simulink model "Perfect_Lineaer"  (R2017a)
settings: Solver=VariableStepAuto  StartTime=0.0  StopTime=17  FixedStep=0.01  RelTol=1e-3
values from neighbouring files (symbols this model uses):
  A = [-4.65E-06	0.0001701	-0.0002836	0	0	0	-2.56E-06	-7.97E-06	3.61E-06 ... (first row only)    [surfaces_setup_test.m]
  A0 = [-4.65E-06	0.0001701	-0.0002836	0	0	0	0	-1.43	0 ... (first row only)    [surfaces_setup_test.m]
  a0_s2345 = [0;0;0.05;0.05]    [HW5_4_surfaces.m]    (also in TEST_aerosetup.m; surfaces_setup_test.m)
  A_2345 = c_2345.*b_2345    [HW5_4_surfaces.m]    (also in TEST_aerosetup.m; surfaces_setup_test.m)
  Aileron_left = 0    [HW5_4_surfaces.m]    (also in TEST_aerosetup.m; surfaces_setup_test.m)
  Aileron_right = 0    [HW5_4_surfaces.m]    (also in TEST_aerosetup.m; surfaces_setup_test.m)
  B = [-7.98E-09	7.83E-09	1.68E-09	2.75E-10 ... (first row only)    [surfaces_setup_test.m]
  B0 = [-6.2	6.2	0	0.45 ... (first row only)    [surfaces_setup_test.m]
  c_2345 = [0.075;0.08;0.1;0.1]    [HW5_4_surfaces.m]    (also in TEST_aerosetup.m; surfaces_setup_test.m)
  CD0_s2345 = [0.01;0.01;0.01;0.01]    [HW5_4_surfaces.m]    (also in TEST_aerosetup.m; surfaces_setup_test.m)
  CDa_s2345 = [1;1;1;1]    [HW5_4_surfaces.m]    (also in TEST_aerosetup.m; surfaces_setup_test.m)
  CL0_2345 = [0;0; 0.05; 0.05]    [HW5_4_surfaces.m]    (also in TEST_aerosetup.m; surfaces_setup_test.m)
  CLa = 2*pi*(r./(2+r))    [HW5_4_surfaces.m]    (also in TEST_aerosetup.m; surfaces_setup_test.m)
  CM0_s2345 = [0;0;-0.05;-0.05]    [HW5_4_surfaces.m]    (also in TEST_aerosetup.m; surfaces_setup_test.m)
  CMa_s2345 = [0; 0; 0; 0]    [HW5_4_surfaces.m]    (also in TEST_aerosetup.m; surfaces_setup_test.m)
  e_s2345 = [0.8;0.8;0.9;0.9]    [HW5_4_surfaces.m]    (also in TEST_aerosetup.m; surfaces_setup_test.m)
  elevator = 0    [HW5_4_surfaces.m]    (also in TEST_aerosetup.m; surfaces_setup_test.m)
  Fext_N = -g_EN * m    [HW5_4_surfaces.m]    (also in TEST_aerosetup.m = [10 10 10]; surfaces_setup_test.m)
  g_EN = [0; 0; 9.81]    [HW5_4_surfaces.m]    (also in TEST_aerosetup.m = [0; 0; 9.8]; surfaces_setup_test.m)
  i_s2345 = [0; 0; 0.05; 0.05;]    [HW5_4_surfaces.m]    (also in TEST_aerosetup.m; surfaces_setup_test.m)
  J_cgp = ones(3)    [surfaces_setup_test.m]
  M_total = sum(MnG(:,1))/1000    [HW5_4_surfaces.m]    (also in TEST_aerosetup.m; surfaces_setup_test.m = sum(MnG1(:,1))/1000)
  Mext_B = [0; 0; 0]    [HW5_4_surfaces.m]    (also in TEST_aerosetup.m = [1; 1; 1]; surfaces_setup_test.m)
  p_E_BE_ini = p_E_BE_ini_deg .* [deg2rad; deg2rad; 1]    [HW5_4_surfaces.m]    (also in TEST_aerosetup.m; surfaces_setup_test.m)
  r = b_2345./c_2345    [HW5_4_surfaces.m]    (also in TEST_aerosetup.m; surfaces_setup_test.m)
  Rearth = 6371000    [HW5_4_surfaces.m]    (also in TEST_aerosetup.m; surfaces_setup_test.m)
  rudder = 0    [HW5_4_surfaces.m]    (also in TEST_aerosetup.m; surfaces_setup_test.m)
  Theta_ini = Theta_ini_deg * deg2rad    [HW5_4_surfaces.m]    (also in TEST_aerosetup.m; surfaces_setup_test.m)
  U0 = [Aileron_right;Aileron_left;elevator;rudder]    [surfaces_setup_test.m]
  v_N_AE = [0;0;0]    [HW5_4_surfaces.m]    (also in TEST_aerosetup.m; surfaces_setup_test.m)
  Vbbe_int = [10; 0; 0]    [HW5_4_surfaces.m]    (also in TEST_aerosetup.m; surfaces_setup_test.m = [5; 0; 0])
  w_B_BE_ini = [1e0; 1e-2; 1e-2]    [HW5_4_surfaces.m]    (also in TEST_aerosetup.m; surfaces_setup_test.m)
  X0 = [w_B_BE_ini;Theta_ini;Vbbe_int]    [surfaces_setup_test.m]
  xyz_s = [[-0.76 0 0.16];[-0.76 0 -0.09];[-0.23 0.44 0];[-0.23 -0.44 0];]    [HW5_4_surfaces.m]    (also in TEST_aerosetup.m; surfaces_setup_test.m)
undefined symbols (not defined in the file or in its folder): Discrete, Earth, K, Time, WGS84
libraries: simulink x83, aerolibfltsims x5, dspsrcs4 x4, simulink_extras x4, dspinverses x3, vrlib x2, sharedtransform x1, aerolibtransform2 x1, aerolibutil x1, sharedutil x1, ctrlSharedLib x1
(part 2 of 8)

== system Perfect_Lineaer/My State Equa_with surf ==
  Band-Limited White Noise : simulink/Sources/Band-Limited White Noise  Cov=[0.1]  Ts=0.1  seed=[23341]
  Colored Noise : dspsrcs4/Colored Noise  Color=white  InverseFrequencyPower=1  NumChannels=1  OutputDataType=double  SamplesPerFrame=1  SampleTime=0.001  RandomStream=mt19937ar with seed  Seed=67  SimulateUsing=Interpreted execution
      settings: SourceProductName=DSP System Toolbox  SourceProductBaseCode=DS
  Demux : Demux  Outputs=3  BusSelectionMode=on
  Demux1 : Demux  Outputs=3
  Demux2 : Demux  Outputs=3
  Gain : Gain
  Gain1 : Gain  Gain=0.05
  Gain2 : Gain  Gain=0.01
  Mux1 : Mux  Inputs=2
  Mux2 : Mux  Inputs=2
  Mux3 : Mux  Inputs=2
  PID Controller : simulink/Continuous/PID Controller  Controller=PID  TimeDomain=Continuous-time  SampleTime=-1  IntegratorMethod=Forward Euler  FilterMethod=Forward Euler  Form=Parallel  UseFilter=on  ControllerParametersSource=internal  P=-1.24371882307401e-06  I=-2.52279405780551e-11  D=-0.0136233397121708  N=0.397355587236386  InitialConditionSource=internal  InitialConditionForIntegrator=0  InitialConditionForFilter=0  ExternalReset=none  LimitOutput=off  UpperSaturationLimit=inf  LowerSaturationLimit=-inf  LinearizeAsGain=on  AntiWindupMode=none  Kb=1  TrackingMode=off  Kt=1  PParamMin=[]  PParamMax=[]  IParamMin=[]  IParamMax=[]  DParamMin=[]  DParamMax=[]  NParamMin=[]  NParamMax=[]  KbParamMin=[]  KbParamMax=[]  KtParamMin=[]  KtParamMax=[]  POutMin=[]  POutMax=[]  IOutMin=[]  IOutMax=[]  DOutMin=[]  DOutMax=[]  NOutMin=[]  NOutMax=[]  KbOutMin=[]  KbOutMax=[]  KtOutMin=[]  KtOutMax=[]  IntegratorOutMin=[]  IntegratorOutMax=[]  FilterOutMin=[]  FilterOutMax=[]  SumOutMin=[]  SumOutMax=[]  SumI1OutMin=[]  SumI1OutMax=[]  SumI2OutMin=[]  SumI2OutMax=[]  SumI3OutMin=[]  SumI3OutMax=[]  SumDOutMin=[]  SumDOutMax=[]  SaturationOutMin=[]  SaturationOutMax=[]  IntegratorContinuousStateAttributes=''  IntegratorStateMustResolveToSignalObject=off  IntegratorRTWStateStorageClass=Auto  FilterContinuousStateAttributes=''  FilterStateMustResolveToSignalObject=off  FilterRTWStateStorageClass=Auto  DifferentiatorICPrevScaledInput=0  DifferentiatorOutMin=[]  DifferentiatorOutMax=[]  InitialConditionSetting=State (most efficient)
  PID Controller1 : simulink/Continuous/PID Controller  Controller=PID  TimeDomain=Continuous-time  SampleTime=-1  IntegratorMethod=Forward Euler  FilterMethod=Forward Euler  Form=Parallel  UseFilter=on  ControllerParametersSource=internal  P=0.206020341004349  I=0.0106225881647426  D=0.887791188699333  N=1010.04325893263  InitialConditionSource=internal  InitialConditionForIntegrator=0  InitialConditionForFilter=0  ExternalReset=none  LimitOutput=off  UpperSaturationLimit=inf  LowerSaturationLimit=-inf  LinearizeAsGain=on  AntiWindupMode=none  Kb=1  TrackingMode=off  Kt=1  PParamMin=[]  PParamMax=[]  IParamMin=[]  IParamMax=[]  DParamMin=[]  DParamMax=[]  NParamMin=[]  NParamMax=[]  KbParamMin=[]  KbParamMax=[]  KtParamMin=[]  KtParamMax=[]  POutMin=[]  POutMax=[]  IOutMin=[]  IOutMax=[]  DOutMin=[]  DOutMax=[]  NOutMin=[]  NOutMax=[]  KbOutMin=[]  KbOutMax=[]  KtOutMin=[]  KtOutMax=[]  IntegratorOutMin=[]  IntegratorOutMax=[]  FilterOutMin=[]  FilterOutMax=[]  SumOutMin=[]  SumOutMax=[]  SumI1OutMin=[]  SumI1OutMax=[]  SumI2OutMin=[]  SumI2OutMax=[]  SumI3OutMin=[]  SumI3OutMax=[]  SumDOutMin=[]  SumDOutMax=[]  SaturationOutMin=[]  SaturationOutMax=[]  IntegratorContinuousStateAttributes=''  IntegratorStateMustResolveToSignalObject=off  IntegratorRTWStateStorageClass=Auto  FilterContinuousStateAttributes=''  FilterStateMustResolveToSignalObject=off  FilterRTWStateStorageClass=Auto  DifferentiatorICPrevScaledInput=0  DifferentiatorOutMin=[]  DifferentiatorOutMax=[]  InitialConditionSetting=State (most efficient)
  PID Controller2 : simulink/Continuous/PID Controller  Controller=PID  TimeDomain=Continuous-time  SampleTime=-1  IntegratorMethod=Forward Euler  FilterMethod=Forward Euler  Form=Parallel  UseFilter=on  ControllerParametersSource=internal  P=0.206020341004349  I=0.0106225881647426  D=0.887791188699333  N=1010.04325893263  InitialConditionSource=internal  InitialConditionForIntegrator=0  InitialConditionForFilter=0  ExternalReset=none  LimitOutput=off  UpperSaturationLimit=inf  LowerSaturationLimit=-inf  LinearizeAsGain=on  AntiWindupMode=none  Kb=1  TrackingMode=off  Kt=1  PParamMin=[]  PParamMax=[]  IParamMin=[]  IParamMax=[]  DParamMin=[]  DParamMax=[]  NParamMin=[]  NParamMax=[]  KbParamMin=[]  KbParamMax=[]  KtParamMin=[]  KtParamMax=[]  POutMin=[]  POutMax=[]  IOutMin=[]  IOutMax=[]  DOutMin=[]  DOutMax=[]  NOutMin=[]  NOutMax=[]  KbOutMin=[]  KbOutMax=[]  KtOutMin=[]  KtOutMax=[]  IntegratorOutMin=[]  IntegratorOutMax=[]  FilterOutMin=[]  FilterOutMax=[]  SumOutMin=[]  SumOutMax=[]  SumI1OutMin=[]  SumI1OutMax=[]  SumI2OutMin=[]  SumI2OutMax=[]  SumI3OutMin=[]  SumI3OutMax=[]  SumDOutMin=[]  SumDOutMax=[]  SaturationOutMin=[]  SaturationOutMax=[]  IntegratorContinuousStateAttributes=''  IntegratorStateMustResolveToSignalObject=off  IntegratorRTWStateStorageClass=Auto  FilterContinuousStateAttributes=''  FilterStateMustResolveToSignalObject=off  FilterRTWStateStorageClass=Auto  DifferentiatorICPrevScaledInput=0  DifferentiatorOutMin=[]  DifferentiatorOutMax=[]  InitialConditionSetting=State (most efficient)
  Scope{,1..4} (5 alike) : Scope
  State-Space (with initial outputs) : simulink_extras/Additional Linear/State-Space (with initial outputs)  A=|  B=[1;1;1;1;1;1;1;1;1]  C=eye(9)  D=[0;0;0;0;0;0;0;0;0]  U0=1  Y0=.5
      | [4.65E-06	0.0003206	-0.0002836	0	0	0	-3.61E-06	-1.11E-05	5.08E-06;
      | -0.0004817	0	0.004483	0	0	0	-0.0009403	0.0007193	-0.001111;
      | 0.0001102	0.001788	-4.65E-06	0	0	0	-4.49E-05	-0.000135	6.27E-05;
      | 1	0.3858	-0.8841	-0.0001586	0.0006637	0	0	0	0;
      | 0	-0.9165	-0.3999	-0.0003438	0	0	0	0	0;
      | 0	0.5557	-1.273	-0.0002285	0.0004608	0	0	0	0;
      | 0	-0.003349	0.002001	-3.476	-2.786	3.102	0.0001527	-0.0002979	-0.0001301;
      | 0.003349	0	0.002582	-30.67	-2.13	30.73	0.0002746	7.64E-05	0.00463;
      | -0.002001	-0.002582	0	-1.42E-10	-22.26	-3.329	0.0001314	-0.004547	-0.0001848
      | ]
      settings: SourceProductName=Simulink  SourceProductBaseCode=SL
  State-Space (with initial outputs)1 : simulink_extras/Additional Linear/State-Space (with initial outputs)  A=|  B=[1;1;1]  C=eye(3)  D=[0;0;0]  U0=1  Y0=.5
      | [0	0.01	0;
      | -0.01	0	0;
      | 0.01	0	0
      | ]
      settings: SourceProductName=Simulink  SourceProductBaseCode=SL
  State-Space (with initial outputs)2 : simulink_extras/Additional Linear/State-Space (with initial outputs)  A=|  B=[1;1;1;1]  C=eye(4)  D=[0;0;0;0]  U0=1  Y0=.5
      | [-0.0025	0.4999	0.004999	0.0025;
      | -0.2475	0	0.004999	0.2475;
      | -0.2524	-0.004999	0	0.2524;
      | -0.0025	0.004999	-0.4999	0.0025
      | ]
      settings: SourceProductName=Simulink  SourceProductBaseCode=SL
  Step1 : Step  Time=5  After=-50  SampleTime=0
  Step2 : Step  Time=5  After=-50  SampleTime=0
  Step3 : Step  Time=5  After=-50  SampleTime=0
  Sum : Sum  Inputs=|+-
  Sum1 : Sum  Inputs=|+++
  Sum2 : Sum  Inputs=|+-
  Sum3 : Sum  Inputs=|+-
  Terminator{,1..5} (6 alike) : Terminator
  wires:
  Step3/1 -> Mux1/2, Sum/1
  Mux1/1 -> Scope1/1
  Sum/1 -> PID Controller/1
  Demux/2 -> Terminator1/1
  Demux/1 -> Terminator/1
  Demux/3 -> Sum1/1, Mux1/1
  State-Space (with initial outputs)/1 -> Scope2/1, Demux/1
  Colored Noise/1 -> Sum1/2
  PID Controller/1 -> State-Space (with initial outputs)/1
  Sum1/1 -> Gain/1
  Gain/1 -> Sum/2, Scope/1
  Band-Limited White Noise/1 -> Sum1/3
  Demux2/1 -> Terminator4/1
  Mux3/1 -> Scope4/1
  Demux2/3 -> Mux3/1, Gain2/1
  State-Space (with initial outputs)1/1 -> Demux1/1
  Mux2/1 -> Scope3/1
  Step2/1 -> Mux2/2, Sum2/1
  Step1/1 -> Mux3/2, Sum3/1
  Sum3/1 -> PID Controller2/1
  Demux1/2 -> Terminator3/1
  Demux1/3 -> Mux2/1, Gain1/1
  Gain2/1 -> Sum3/2
  Demux2/2 -> Terminator5/1
  PID Controller2/1 -> State-Space (with initial outputs)2/1
  Gain1/1 -> Sum2/2
  PID Controller1/1 -> State-Space (with initial outputs)1/1
  Sum2/1 -> PID Controller1/1
  Demux1/1 -> Terminator2/1
  State-Space (with initial outputs)2/1 -> Demux2/1

== system Perfect_Lineaer/Perfect_State Equa ==
  note: Inner loop
  note: Outer loop
  note: State loop
  A0 : Gain  Gain=A0  Multiplication=Matrix(K*u)
  B0 : Gain  Gain=B0  Multiplication=Matrix(K*u)
  Band-Limited White Noise : simulink/Sources/Band-Limited White Noise  Commented=on  Cov=[0.1]  Ts=0.1  seed=[23341]
  Colored Noise : dspsrcs4/Colored Noise  Commented=on  Color=white  InverseFrequencyPower=1  NumChannels=1  OutputDataType=double  SamplesPerFrame=1  SampleTime=0.001  RandomStream=mt19937ar with seed  Seed=67  SimulateUsing=Interpreted execution
      settings: SourceProductName=DSP System Toolbox  SourceProductBaseCode=DS
  Constant : Constant  Value=U0
  Constant1 : Constant  Value=X0
  Integrator : Integrator  InitialConditionSource=external
  Kd Based on Rlocus : Gain  Multiplication=Matrix(K*u)
  Kp for speed control : Gain  Commented=on
  PID Controller : simulink/Continuous/PID Controller  Controller=PID  TimeDomain=Continuous-time  SampleTime=-1  IntegratorMethod=Forward Euler  FilterMethod=Forward Euler  Form=Parallel  UseFilter=on  ControllerParametersSource=internal  P=10  I=0  D=0  N=100  InitialConditionSource=internal  InitialConditionForIntegrator=0  InitialConditionForFilter=0  ExternalReset=none  LimitOutput=off  UpperSaturationLimit=inf  LowerSaturationLimit=-inf  LinearizeAsGain=on  AntiWindupMode=none  Kb=1  TrackingMode=off  Kt=1  PParamMin=[]  PParamMax=[]  IParamMin=[]  IParamMax=[]  DParamMin=[]  DParamMax=[]  NParamMin=[]  NParamMax=[]  KbParamMin=[]  KbParamMax=[]  KtParamMin=[]  KtParamMax=[]  POutMin=[]  POutMax=[]  IOutMin=[]  IOutMax=[]  DOutMin=[]  DOutMax=[]  NOutMin=[]  NOutMax=[]  KbOutMin=[]  KbOutMax=[]  KtOutMin=[]  KtOutMax=[]  IntegratorOutMin=[]  IntegratorOutMax=[]  FilterOutMin=[]  FilterOutMax=[]  SumOutMin=[]  SumOutMax=[]  SumI1OutMin=[]  SumI1OutMax=[]  SumI2OutMin=[]  SumI2OutMax=[]  SumI3OutMin=[]  SumI3OutMax=[]  SumDOutMin=[]  SumDOutMax=[]  SaturationOutMin=[]  SaturationOutMax=[]  IntegratorContinuousStateAttributes=''  IntegratorStateMustResolveToSignalObject=off  IntegratorRTWStateStorageClass=Auto  FilterContinuousStateAttributes=''  FilterStateMustResolveToSignalObject=off  FilterRTWStateStorageClass=Auto  DifferentiatorICPrevScaledInput=0  DifferentiatorOutMin=[]  DifferentiatorOutMax=[]  InitialConditionSetting=State (most efficient)
  Scope : Scope
  Sum : Sum  Inputs=|++
  Sum1 : Sum  Inputs=|+-
  Sum2 : Sum  Commented=on  Inputs=|+-
  Sum3 : Sum  Commented=on  Inputs=|+++
  wires:
  A0/1 -> Sum/2
  Constant1/1 -> Integrator/2
  Sum/1 -> Integrator/1
  B0/1 -> Sum1/1
  Kd Based on Rlocus/1 -> Sum1/2
  Sum3/1 -> Kp for speed control/1
  Integrator/1 -> Sum3/1, Kd Based on Rlocus/1, Scope/1, A0/1
  Band-Limited White Noise/1 -> Sum3/3
  Kp for speed control/1 -> Sum2/2
  Colored Noise/1 -> Sum3/2
  Constant/1 -> B0/1
  Sum1/1 -> PID Controller/1
  PID Controller/1 -> Sum/1

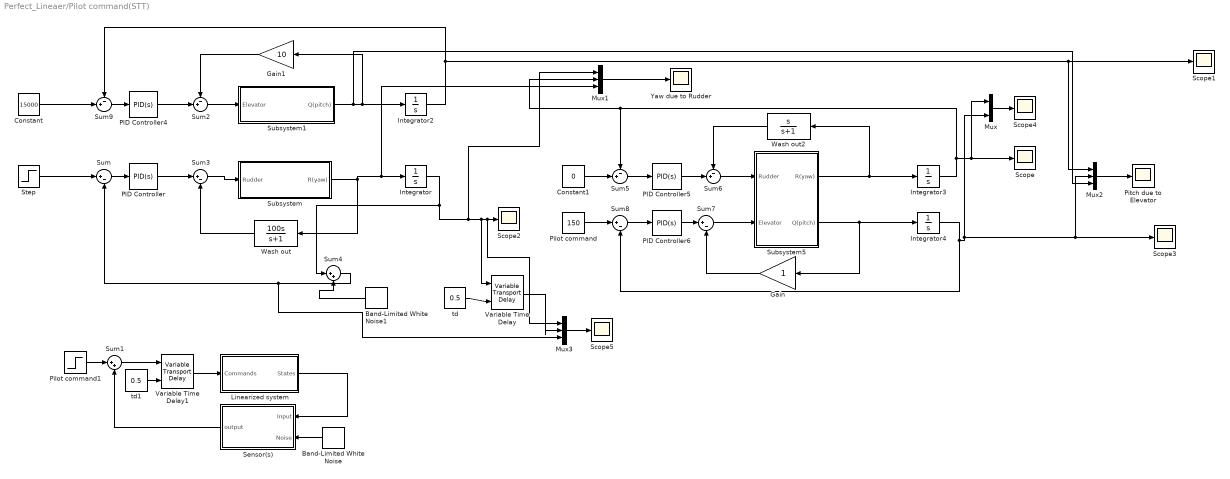
== system Perfect_Lineaer/Pilot command(STT) ==
  Band-Limited White Noise : simulink/Sources/Band-Limited White Noise  Cov=[0.1]  Ts=0.1  seed=[23341]
  Band-Limited White Noise1 : simulink/Sources/Band-Limited White Noise  Cov=[0.01]  Ts=0.8  seed=[25]
  Constant : Constant  Value=15000
  Constant1 : Constant  Value=0
  Gain : Gain
  Gain1 : Gain  Gain=10
  Integrator{,2..4} (4 alike) : Integrator
  Linearized system : Subsystem
  Mux : Mux  Inputs=2
  Mux1 : Mux  Inputs=3
  Mux2 : Mux  Inputs=3
  Mux3 : Mux  Inputs=3
  PID Controller : simulink/Continuous/PID Controller  Controller=PID  TimeDomain=Continuous-time  SampleTime=-1  IntegratorMethod=Forward Euler  FilterMethod=Forward Euler  Form=Parallel  UseFilter=on  ControllerParametersSource=internal  P=1000  I=0  D=1  N=100  InitialConditionSource=internal  InitialConditionForIntegrator=0  InitialConditionForFilter=0  ExternalReset=none  LimitOutput=off  UpperSaturationLimit=inf  LowerSaturationLimit=-inf  LinearizeAsGain=on  AntiWindupMode=none  Kb=1  TrackingMode=off  Kt=1  PParamMin=[]  PParamMax=[]  IParamMin=[]  IParamMax=[]  DParamMin=[]  DParamMax=[]  NParamMin=[]  NParamMax=[]  KbParamMin=[]  KbParamMax=[]  KtParamMin=[]  KtParamMax=[]  POutMin=[]  POutMax=[]  IOutMin=[]  IOutMax=[]  DOutMin=[]  DOutMax=[]  NOutMin=[]  NOutMax=[]  KbOutMin=[]  KbOutMax=[]  KtOutMin=[]  KtOutMax=[]  IntegratorOutMin=[]  IntegratorOutMax=[]  FilterOutMin=[]  FilterOutMax=[]  SumOutMin=[]  SumOutMax=[]  SumI1OutMin=[]  SumI1OutMax=[]  SumI2OutMin=[]  SumI2OutMax=[]  SumI3OutMin=[]  SumI3OutMax=[]  SumDOutMin=[]  SumDOutMax=[]  SaturationOutMin=[]  SaturationOutMax=[]  IntegratorContinuousStateAttributes=''  IntegratorStateMustResolveToSignalObject=off  IntegratorRTWStateStorageClass=Auto  FilterContinuousStateAttributes=''  FilterStateMustResolveToSignalObject=off  FilterRTWStateStorageClass=Auto  DifferentiatorICPrevScaledInput=0  DifferentiatorOutMin=[]  DifferentiatorOutMax=[]  InitialConditionSetting=State (most efficient)
  PID Controller4 : simulink/Continuous/PID Controller  Controller=PID  TimeDomain=Continuous-time  SampleTime=-1  IntegratorMethod=Forward Euler  FilterMethod=Forward Euler  Form=Parallel  UseFilter=on  ControllerParametersSource=internal  P=1000  I=0  D=0  N=100  InitialConditionSource=internal  InitialConditionForIntegrator=0  InitialConditionForFilter=0  ExternalReset=none  LimitOutput=off  UpperSaturationLimit=inf  LowerSaturationLimit=-inf  LinearizeAsGain=on  AntiWindupMode=none  Kb=1  TrackingMode=off  Kt=1  PParamMin=[]  PParamMax=[]  IParamMin=[]  IParamMax=[]  DParamMin=[]  DParamMax=[]  NParamMin=[]  NParamMax=[]  KbParamMin=[]  KbParamMax=[]  KtParamMin=[]  KtParamMax=[]  POutMin=[]  POutMax=[]  IOutMin=[]  IOutMax=[]  DOutMin=[]  DOutMax=[]  NOutMin=[]  NOutMax=[]  KbOutMin=[]  KbOutMax=[]  KtOutMin=[]  KtOutMax=[]  IntegratorOutMin=[]  IntegratorOutMax=[]  FilterOutMin=[]  FilterOutMax=[]  SumOutMin=[]  SumOutMax=[]  SumI1OutMin=[]  SumI1OutMax=[]  SumI2OutMin=[]  SumI2OutMax=[]  SumI3OutMin=[]  SumI3OutMax=[]  SumDOutMin=[]  SumDOutMax=[]  SaturationOutMin=[]  SaturationOutMax=[]  IntegratorContinuousStateAttributes=''  IntegratorStateMustResolveToSignalObject=off  IntegratorRTWStateStorageClass=Auto  FilterContinuousStateAttributes=''  FilterStateMustResolveToSignalObject=off  FilterRTWStateStorageClass=Auto  DifferentiatorICPrevScaledInput=0  DifferentiatorOutMin=[]  DifferentiatorOutMax=[]  InitialConditionSetting=State (most efficient)
  PID Controller5 : simulink/Continuous/PID Controller  Controller=PID  TimeDomain=Continuous-time  SampleTime=-1  IntegratorMethod=Forward Euler  FilterMethod=Forward Euler  Form=Parallel  UseFilter=on  ControllerParametersSource=internal  P=1000  I=0  D=1  N=100  InitialConditionSource=internal  InitialConditionForIntegrator=0  InitialConditionForFilter=0  ExternalReset=none  LimitOutput=off  UpperSaturationLimit=inf  LowerSaturationLimit=-inf  LinearizeAsGain=on  AntiWindupMode=none  Kb=1  TrackingMode=off  Kt=1  PParamMin=[]  PParamMax=[]  IParamMin=[]  IParamMax=[]  DParamMin=[]  DParamMax=[]  NParamMin=[]  NParamMax=[]  KbParamMin=[]  KbParamMax=[]  KtParamMin=[]  KtParamMax=[]  POutMin=[]  POutMax=[]  IOutMin=[]  IOutMax=[]  DOutMin=[]  DOutMax=[]  NOutMin=[]  NOutMax=[]  KbOutMin=[]  KbOutMax=[]  KtOutMin=[]  KtOutMax=[]  IntegratorOutMin=[]  IntegratorOutMax=[]  FilterOutMin=[]  FilterOutMax=[]  SumOutMin=[]  SumOutMax=[]  SumI1OutMin=[]  SumI1OutMax=[]  SumI2OutMin=[]  SumI2OutMax=[]  SumI3OutMin=[]  SumI3OutMax=[]  SumDOutMin=[]  SumDOutMax=[]  SaturationOutMin=[]  SaturationOutMax=[]  IntegratorContinuousStateAttributes=''  IntegratorStateMustResolveToSignalObject=off  IntegratorRTWStateStorageClass=Auto  FilterContinuousStateAttributes=''  FilterStateMustResolveToSignalObject=off  FilterRTWStateStorageClass=Auto  DifferentiatorICPrevScaledInput=0  DifferentiatorOutMin=[]  DifferentiatorOutMax=[]  InitialConditionSetting=State (most efficient)
  PID Controller6 : simulink/Continuous/PID Controller  Controller=PID  TimeDomain=Continuous-time  SampleTime=-1  IntegratorMethod=Forward Euler  FilterMethod=Forward Euler  Form=Parallel  UseFilter=on  ControllerParametersSource=internal  P=1000  I=0  D=0  N=100  InitialConditionSource=internal  InitialConditionForIntegrator=0  InitialConditionForFilter=0  ExternalReset=none  LimitOutput=off  UpperSaturationLimit=inf  LowerSaturationLimit=-inf  LinearizeAsGain=on  AntiWindupMode=none  Kb=1  TrackingMode=off  Kt=1  PParamMin=[]  PParamMax=[]  IParamMin=[]  IParamMax=[]  DParamMin=[]  DParamMax=[]  NParamMin=[]  NParamMax=[]  KbParamMin=[]  KbParamMax=[]  KtParamMin=[]  KtParamMax=[]  POutMin=[]  POutMax=[]  IOutMin=[]  IOutMax=[]  DOutMin=[]  DOutMax=[]  NOutMin=[]  NOutMax=[]  KbOutMin=[]  KbOutMax=[]  KtOutMin=[]  KtOutMax=[]  IntegratorOutMin=[]  IntegratorOutMax=[]  FilterOutMin=[]  FilterOutMax=[]  SumOutMin=[]  SumOutMax=[]  SumI1OutMin=[]  SumI1OutMax=[]  SumI2OutMin=[]  SumI2OutMax=[]  SumI3OutMin=[]  SumI3OutMax=[]  SumDOutMin=[]  SumDOutMax=[]  SaturationOutMin=[]  SaturationOutMax=[]  IntegratorContinuousStateAttributes=''  IntegratorStateMustResolveToSignalObject=off  IntegratorRTWStateStorageClass=Auto  FilterContinuousStateAttributes=''  FilterStateMustResolveToSignalObject=off  FilterRTWStateStorageClass=Auto  DifferentiatorICPrevScaledInput=0  DifferentiatorOutMin=[]  DifferentiatorOutMax=[]  InitialConditionSetting=State (most efficient)
  Pilot command : Constant  Value=150
  Pilot command1 : Step  After=20000  SampleTime=0
  Pitch due to Elevator : Scope
  Scope{,1..5} (6 alike) : Scope
  Sensor(s) : Subsystem
  Step : Step  After=20000  SampleTime=0
  Subsystem : Subsystem
  Subsystem1 : Subsystem
  Subsystem5 : Subsystem
  Sum{,3,7..8} (4 alike) : Sum  Inputs=|+-
  Sum1 : Sum  Inputs=|++
  Sum{2,5..6,9} (4 alike) : Sum  Inputs=-+|
  Sum4 : Sum  Inputs=|++
  Variable Time Delay : VariableTransportDelay  VariableDelayType=Variable transport delay  MaximumDelay=10
  Variable Time Delay1 : VariableTransportDelay  VariableDelayType=Variable transport delay  MaximumDelay=10
  Wash out : TransferFcn  Numerator=[100 0]  Denominator=[1 1]
  Wash out2 : TransferFcn  Numerator=[1 0]  Denominator=[1 1]
  Yaw due to Rudder : Scope
  td : Constant  Value=0.5
  td1 : Constant  Value=0.5
  wires:
  Wash out/1 -> Sum3/2
  Sum6/1 -> Subsystem5/1(Rudder)
  Integrator/1 -> Sum4/1, Variable Time Delay/1, Mux3/1, Scope2/1, Mux1/1
  Wash out2/1 -> Sum6/1
  Subsystem5/1(R(yaw)) -> Integrator3/1, Wash out2/1
  PID Controller5/1 -> Sum6/2
  Integrator3/1 -> Sum5/1, Mux1/2, Scope/1, Mux/1
  Sum/1 -> PID Controller/1
  PID Controller/1 -> Sum3/1
  Subsystem/1(R(yaw)) -> Integrator/1, Mux1/3, Wash out/1
  Subsystem5/2(Q(pitch)) -> Integrator4/1, Gain/1
  Sum7/1 -> Subsystem5/2(Elevator)
  Subsystem1/1(Q(pitch)) -> Mux2/3, Integrator2/1, Gain1/1
  Sum9/1 -> PID Controller4/1
  Sum5/1 -> PID Controller5/1
  Gain/1 -> Sum7/2
  Sum2/1 -> Subsystem1/1(Elevator)
  Constant/1 -> Sum9/2
  Sum3/1 -> Subsystem/1(Rudder)
  Mux2/1 -> Pitch due to Elevator/1
  Integrator2/1 -> Scope1/1, Mux2/1, Sum9/1
  Constant1/1 -> Sum5/2
  PID Controller6/1 -> Sum7/1
  Gain1/1 -> Sum2/1
  Step/1 -> Sum/1
  PID Controller4/1 -> Sum2/2
  Integrator4/1 -> Mux/2, Scope3/1, Mux2/2, Sum8/2
  Mux/1 -> Scope4/1
  Sum8/1 -> PID Controller6/1
  Pilot command/1 -> Sum8/1
  Mux1/1 -> Yaw due to Rudder/1
  td/1 -> Variable Time Delay/2
  Variable Time Delay/1 -> Mux3/2
  Mux3/1 -> Scope5/1
  Variable Time Delay1/1 -> Linearized system/1(Commands)
  td1/1 -> Variable Time Delay1/2
  Pilot command1/1 -> Sum1/1
  Linearized system/1(States) -> Sensor(s)/1(Input)
  Sensor(s)/1(output) -> Sum1/2
  Sum1/1 -> Variable Time Delay1/1
  Band-Limited White Noise/1 -> Sensor(s)/2(Noise)
  Sum4/1 -> Mux3/3, Sum/2
  Band-Limited White Noise1/1 -> Sum4/2

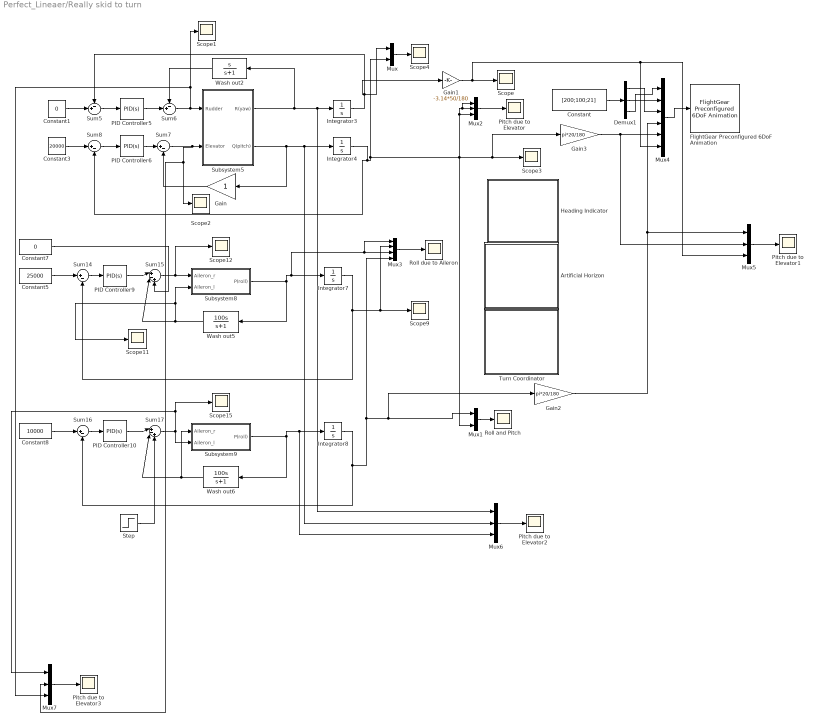
== system Perfect_Lineaer/Really skid to turn ==
  Artificial Horizon : Subsystem  DialogController=aeroblksHMICreateDDGDialog  IsWebBlock=on  mask(MWDashboardBlock){webBlockId=d62fc3a9-950b-49b7-8093-1c4fc0d2cd0d, webBlockType=artificialhorizon, ShowInLibBrowser=on, ShowInitialText=on, HMISrcModelName=Perfect_Lineaer}
      mask prompts: webBlockId "WebBlock Id"; webBlockType "WebBlock Type"; HMISrcModelName "Source Model"
      mask help: aeroblksHMI:aeroblkhmi:ArtificialHorizonDialogDesc
      mask Help: eval('asbhmihelp(''artificialhorizon'')');
      mask Display:
      | if strcmp(get_param(bdroot(gcb),'BlockDiagramType'), 'library')
      |  image([(matlabroot) '/toolbox/aeroblks/aeroblks/hmi/icons/ArtificialHorizonIcon.svg'])
      | end
  Constant : Constant  Value=[200;100;21]
  Constant1 : Constant  Value=0
  Constant3 : Constant  Value=20000
  Constant5 : Constant  Value=25000
  Constant7 : Constant  Value=0
  Constant8 : Constant  Value=10000
  Demux1 : Demux  Outputs=3
  FlightGear Preconfigured 6DoF Animation : aerolibfltsims/FlightGear Preconfigured 6DoF Animation  xFlightGearVersion=v3.0  DestinationIpAddress=127.0.0.1  DestinationPort=5502  SampleTime=1/30
      settings: SourceProductName=Aerospace Blockset
  Gain : Gain
  Gain1 : Gain  Gain=-3.14*50/180
  Gain2 : Gain  Gain=pi*20/180
  Gain3 : Gain  Gain=pi*20/180
  Heading Indicator : Subsystem  DialogController=aeroblksHMICreateDDGDialog  IsWebBlock=on  mask(MWDashboardBlock){webBlockId=af126bab-eee7-42e1-a5ca-bf7ae56a8065, webBlockType=headingindicator, ShowInLibBrowser=on, ShowInitialText=on, HMISrcModelName=Perfect_Lineaer}
      mask prompts: webBlockId "WebBlock Id"; webBlockType "WebBlock Type"; HMISrcModelName "Source Model"
      mask help: aeroblksHMI:aeroblkhmi:HeadingIndicatorDialogDesc
      mask Help: eval('asbhmihelp(''headingindicator'')');
      mask Display:
      | if strcmp(get_param(bdroot(gcb),'BlockDiagramType'), 'library')
      |  image([(matlabroot) '/toolbox/aeroblks/aeroblks/hmi/icons/HeadingIndicatorIcon.svg'])
      | end
  Integrator{3..4,7..8} (4 alike) : Integrator
  Mux : Mux  Inputs=2
  Mux1 : Mux  Inputs=2
  Mux{2,5..7} (4 alike) : Mux  Inputs=3
  Mux3 : Mux
  Mux4 : Mux  Inputs=6
  PID Controller10 : simulink/Continuous/PID Controller  Controller=PID  TimeDomain=Continuous-time  SampleTime=-1  IntegratorMethod=Forward Euler  FilterMethod=Forward Euler  Form=Parallel  UseFilter=on  ControllerParametersSource=internal  P=1000  I=0  D=0  N=100  InitialConditionSource=internal  InitialConditionForIntegrator=0  InitialConditionForFilter=0  ExternalReset=none  LimitOutput=off  UpperSaturationLimit=inf  LowerSaturationLimit=-inf  LinearizeAsGain=on  AntiWindupMode=none  Kb=1  TrackingMode=off  Kt=1  PParamMin=[]  PParamMax=[]  IParamMin=[]  IParamMax=[]  DParamMin=[]  DParamMax=[]  NParamMin=[]  NParamMax=[]  KbParamMin=[]  KbParamMax=[]  KtParamMin=[]  KtParamMax=[]  POutMin=[]  POutMax=[]  IOutMin=[]  IOutMax=[]  DOutMin=[]  DOutMax=[]  NOutMin=[]  NOutMax=[]  KbOutMin=[]  KbOutMax=[]  KtOutMin=[]  KtOutMax=[]  IntegratorOutMin=[]  IntegratorOutMax=[]  FilterOutMin=[]  FilterOutMax=[]  SumOutMin=[]  SumOutMax=[]  SumI1OutMin=[]  SumI1OutMax=[]  SumI2OutMin=[]  SumI2OutMax=[]  SumI3OutMin=[]  SumI3OutMax=[]  SumDOutMin=[]  SumDOutMax=[]  SaturationOutMin=[]  SaturationOutMax=[]  IntegratorContinuousStateAttributes=''  IntegratorStateMustResolveToSignalObject=off  IntegratorRTWStateStorageClass=Auto  FilterContinuousStateAttributes=''  FilterStateMustResolveToSignalObject=off  FilterRTWStateStorageClass=Auto  DifferentiatorICPrevScaledInput=0  DifferentiatorOutMin=[]  DifferentiatorOutMax=[]  InitialConditionSetting=State (most efficient)
  PID Controller5 : simulink/Continuous/PID Controller  Controller=PID  TimeDomain=Continuous-time  SampleTime=-1  IntegratorMethod=Forward Euler  FilterMethod=Forward Euler  Form=Parallel  UseFilter=on  ControllerParametersSource=internal  P=1000  I=0  D=1  N=100  InitialConditionSource=internal  InitialConditionForIntegrator=0  InitialConditionForFilter=0  ExternalReset=none  LimitOutput=off  UpperSaturationLimit=inf  LowerSaturationLimit=-inf  LinearizeAsGain=on  AntiWindupMode=none  Kb=1  TrackingMode=off  Kt=1  PParamMin=[]  PParamMax=[]  IParamMin=[]  IParamMax=[]  DParamMin=[]  DParamMax=[]  NParamMin=[]  NParamMax=[]  KbParamMin=[]  KbParamMax=[]  KtParamMin=[]  KtParamMax=[]  POutMin=[]  POutMax=[]  IOutMin=[]  IOutMax=[]  DOutMin=[]  DOutMax=[]  NOutMin=[]  NOutMax=[]  KbOutMin=[]  KbOutMax=[]  KtOutMin=[]  KtOutMax=[]  IntegratorOutMin=[]  IntegratorOutMax=[]  FilterOutMin=[]  FilterOutMax=[]  SumOutMin=[]  SumOutMax=[]  SumI1OutMin=[]  SumI1OutMax=[]  SumI2OutMin=[]  SumI2OutMax=[]  SumI3OutMin=[]  SumI3OutMax=[]  SumDOutMin=[]  SumDOutMax=[]  SaturationOutMin=[]  SaturationOutMax=[]  IntegratorContinuousStateAttributes=''  IntegratorStateMustResolveToSignalObject=off  IntegratorRTWStateStorageClass=Auto  FilterContinuousStateAttributes=''  FilterStateMustResolveToSignalObject=off  FilterRTWStateStorageClass=Auto  DifferentiatorICPrevScaledInput=0  DifferentiatorOutMin=[]  DifferentiatorOutMax=[]  InitialConditionSetting=State (most efficient)
  PID Controller6 : simulink/Continuous/PID Controller  Controller=PID  TimeDomain=Continuous-time  SampleTime=-1  IntegratorMethod=Forward Euler  FilterMethod=Forward Euler  Form=Parallel  UseFilter=on  ControllerParametersSource=internal  P=1000  I=0  D=0  N=100  InitialConditionSource=internal  InitialConditionForIntegrator=0  InitialConditionForFilter=0  ExternalReset=none  LimitOutput=off  UpperSaturationLimit=inf  LowerSaturationLimit=-inf  LinearizeAsGain=on  AntiWindupMode=none  Kb=1  TrackingMode=off  Kt=1  PParamMin=[]  PParamMax=[]  IParamMin=[]  IParamMax=[]  DParamMin=[]  DParamMax=[]  NParamMin=[]  NParamMax=[]  KbParamMin=[]  KbParamMax=[]  KtParamMin=[]  KtParamMax=[]  POutMin=[]  POutMax=[]  IOutMin=[]  IOutMax=[]  DOutMin=[]  DOutMax=[]  NOutMin=[]  NOutMax=[]  KbOutMin=[]  KbOutMax=[]  KtOutMin=[]  KtOutMax=[]  IntegratorOutMin=[]  IntegratorOutMax=[]  FilterOutMin=[]  FilterOutMax=[]  SumOutMin=[]  SumOutMax=[]  SumI1OutMin=[]  SumI1OutMax=[]  SumI2OutMin=[]  SumI2OutMax=[]  SumI3OutMin=[]  SumI3OutMax=[]  SumDOutMin=[]  SumDOutMax=[]  SaturationOutMin=[]  SaturationOutMax=[]  IntegratorContinuousStateAttributes=''  IntegratorStateMustResolveToSignalObject=off  IntegratorRTWStateStorageClass=Auto  FilterContinuousStateAttributes=''  FilterStateMustResolveToSignalObject=off  FilterRTWStateStorageClass=Auto  DifferentiatorICPrevScaledInput=0  DifferentiatorOutMin=[]  DifferentiatorOutMax=[]  InitialConditionSetting=State (most efficient)
  PID Controller9 : simulink/Continuous/PID Controller  Controller=PID  TimeDomain=Continuous-time  SampleTime=-1  IntegratorMethod=Forward Euler  FilterMethod=Forward Euler  Form=Parallel  UseFilter=on  ControllerParametersSource=internal  P=100  I=0  D=0  N=100  InitialConditionSource=internal  InitialConditionForIntegrator=0  InitialConditionForFilter=0  ExternalReset=none  LimitOutput=off  UpperSaturationLimit=inf  LowerSaturationLimit=-inf  LinearizeAsGain=on  AntiWindupMode=none  Kb=1  TrackingMode=off  Kt=1  PParamMin=[]  PParamMax=[]  IParamMin=[]  IParamMax=[]  DParamMin=[]  DParamMax=[]  NParamMin=[]  NParamMax=[]  KbParamMin=[]  KbParamMax=[]  KtParamMin=[]  KtParamMax=[]  POutMin=[]  POutMax=[]  IOutMin=[]  IOutMax=[]  DOutMin=[]  DOutMax=[]  NOutMin=[]  NOutMax=[]  KbOutMin=[]  KbOutMax=[]  KtOutMin=[]  KtOutMax=[]  IntegratorOutMin=[]  IntegratorOutMax=[]  FilterOutMin=[]  FilterOutMax=[]  SumOutMin=[]  SumOutMax=[]  SumI1OutMin=[]  SumI1OutMax=[]  SumI2OutMin=[]  SumI2OutMax=[]  SumI3OutMin=[]  SumI3OutMax=[]  SumDOutMin=[]  SumDOutMax=[]  SaturationOutMin=[]  SaturationOutMax=[]  IntegratorContinuousStateAttributes=''  IntegratorStateMustResolveToSignalObject=off  IntegratorRTWStateStorageClass=Auto  FilterContinuousStateAttributes=''  FilterStateMustResolveToSignalObject=off  FilterRTWStateStorageClass=Auto  DifferentiatorICPrevScaledInput=0  DifferentiatorOutMin=[]  DifferentiatorOutMax=[]  InitialConditionSetting=State (most efficient)
  Pitch due to Elevator{,1..3} (4 alike) : Scope
  Roll and Pitch : Scope
  Roll due to Aileron : Scope
  Scope{,1..4,9,11..12,15} (9 alike) : Scope
  Step : Step  Time=8  After=0  SampleTime=0
  Subsystem5 : Subsystem
  Subsystem8 : Subsystem
  Subsystem9 : Subsystem
  Sum{7..8,14,16} (4 alike) : Sum  Inputs=|+-
  Sum15 : Sum  Inputs=|+-+
  Sum17 : Sum  Inputs=|+-+
  Sum5 : Sum  Inputs=-+|
  Sum6 : Sum  Inputs=-+|
  Turn Coordinator : Subsystem  DialogController=aeroblksHMICreateDDGDialog  IsWebBlock=on  mask(MWDashboardBlock){webBlockId=137e4400-b6b5-49ac-a30a-fb68a8b5ca91, webBlockType=turncoordinator, ShowInLibBrowser=on, ShowInitialText=on, HMISrcModelName=Perfect_Lineaer}
      mask prompts: webBlockId "WebBlock Id"; webBlockType "WebBlock Type"; HMISrcModelName "Source Model"
      mask help: aeroblksHMI:aeroblkhmi:TurnCoordinatorDialogDesc
      mask Help: eval('asbhmihelp(''turncoordinator'')');
      mask Display:
      | if strcmp(get_param(bdroot(gcb),'BlockDiagramType'), 'library')
      |  image([(matlabroot) '/toolbox/aeroblks/aeroblks/hmi/icons/TurnCoordinatorIcon.svg'])
      | end
  Wash out2 : TransferFcn  Numerator=[1 0]  Denominator=[1 1]
  Wash out5 : TransferFcn  Numerator=[100 0]  Denominator=[1 1]
  Wash out6 : TransferFcn  Numerator=[100 0]  Denominator=[1 1]
  wires:
  Sum6/1 -> Mux7/3, Scope1/1, Subsystem5/1(Rudder)
  Wash out2/1 -> Sum6/1
  PID Controller5/1 -> Sum6/2
  Integrator3/1 -> Mux/1, Gain1/1, Sum5/1
  Sum5/1 -> PID Controller5/1
  Gain/1 -> Sum7/2
  Mux2/1 -> Pitch due to Elevator/1
  Constant1/1 -> Sum5/2
  PID Controller6/1 -> Sum7/1
  Mux/1 -> Scope4/1
  Sum8/1 -> PID Controller6/1
  Constant3/1 -> Sum8/1
  Sum16/1 -> PID Controller10/1
  Sum14/1 -> PID Controller9/1
  Mux3/1 -> Roll due to Aileron/1
  Wash out6/1 -> Sum17/2, Subsystem9/1(Aileron_r)
  PID Controller10/1 -> Sum17/1
  Integrator7/1 -> Mux3/2, Scope9/1, Sum14/2
  Constant7/1 -> Sum15/3
  Sum15/1 -> Subsystem8/1(Aileron_r), Scope12/1
  Constant5/1 -> Sum14/1
  Subsystem8/1(P(roll)) -> Wash out5/1, Mux3/1, Mux3/3, Integrator7/1
  Wash out5/1 -> Sum15/2, Subsystem8/2(Aileron_l), Scope11/1
  Sum17/1 -> Mux7/1, Scope15/1, Subsystem9/2(Aileron_l)
  PID Controller9/1 -> Sum15/1
  Constant8/1 -> Sum16/1
  Mux1/1 -> Roll and Pitch/1
  Demux1/2 -> Mux4/2
  Demux1/3 -> Mux4/1
  Demux1/1 -> Mux4/3
  Integrator4/1 -> Mux/2, Mux1/2, Gain3/1, Scope3/1, Mux2/3, Mux2/1, Mux2/2, Sum8/2
  Integrator8/1 -> Sum16/2, Gain2/1, Mux1/1, Mux3/4
  Constant/1 -> Demux1/1
  Gain1/1 -> Mux5/3, Mux4/6, Scope/1
  Mux4/1 -> FlightGear Preconfigured 6DoF Animation/1
  Gain2/1 -> Mux4/4, Mux5/1
  Mux5/1 -> Pitch due to Elevator1/1
  Gain3/1 -> Mux5/2, Mux4/5
  Step/1 -> Sum17/3
  Subsystem9/1(P(roll)) -> Wash out6/1, Mux6/3, Integrator8/1
  Mux6/1 -> Pitch due to Elevator2/1
  Subsystem5/1(R(yaw)) -> Mux6/1, Integrator3/1, Wash out2/1
  Subsystem5/2(Q(pitch)) -> Mux6/2, Integrator4/1, Gain/1
  Mux7/1 -> Pitch due to Elevator3/1
  Sum7/1 -> Mux7/2, Scope2/1, Subsystem5/2(Elevator)
